simulink library "commdigbbnd"  (Simulink 5.0)
undefined symbols (not defined in the file or in its folder): j
libraries: commanabbnd x8, commutil x5, commdigbbnd x2
settings Model: Creator=tdelve  LastModifiedBy=mmclerno

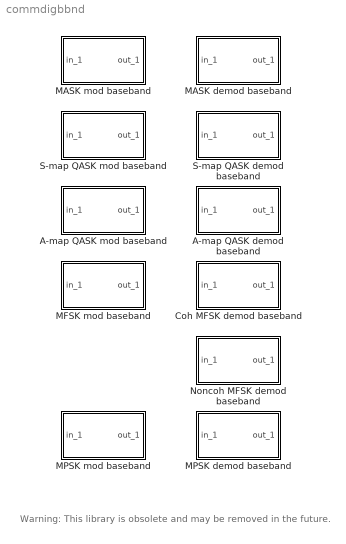
== system commdigbbnd ==
  note: Warning:  This library is obsolete and may be
      | removed in the future.
  A-map QASK demod baseband : Subsystem  mask(Baseband A-QASK demodulation){y1=real(exp(j*[0:16-1]/16*pi*2)), y2=imag(exp(j*[0:16-1]/16*pi*2)), td=0.1, num=[1;1], Ph=0, ts=0.001}
      mask prompts: y1 "Constellation in-phase component:"; y2 "Constellation quadrature component:"; td "Symbol interval and offset (sec):"; num "Lowpass filter [num; den], a 2 row matrix:"; Ph "Initial phase (rad):"; ts "Sample time (sec):"
      mask help: Demodulate the complex envelope of a QASK modulated signal. The arbitrary constellation is defined by in-phase and quadrature vectors.
      mask init:
      | den=num(2,:);num=num(1,:);
      mask Help: This block demodulates the complex envelope of a QASK modulated signal with user-defined arbitrary constellation. The vector length of the in-phase and quadrature components vectors should have the same length. The outputs are integers in the range [0, M-1], where M is the vector length of in-phase or quadrature. When the symbol interval is a two-element vector, the second element is the offset (default 0).
      mask Display:
      | plot(0,0,100,100,[5+1.5*[[0:.8:10] [10 20] [20:.8:30]] 50 50 50 50+15*[0 1 1 2 2 3]],[85+10*[sin([0:.8:10]*pi*2/5) 0 0 sin([20:.8:30]*pi*2/5)] 85 99 75 85+8*[1 1 -1 -1 1 1]]);
      | disp('A-QASK')
  A-map QASK mod baseband : Subsystem  mask(Baseband A-QASK modulation){y1=real(exp(j*[0:16-1]/16*pi*2)), y2=imag(exp(j*[0:16-1]/16*pi*2)), td=0.1, Ph=0, ts=0.001}
      mask prompts: y1 "Constellation in-phase component:"; y2 "Constellation quadrature component:"; td "Input symbol interval and offset (sec):"; Ph "Initial phase (rad):"; ts "Sample time (sec):"
      mask help: Output the complex envelope of QASK modulation. The arbitrary constellation is defined by in-phase and quadrature vectors.
      mask Help: This block outputs the complex envelope of a QASK modulated signal with user-defined arbitrary constellation. The vector length of the in-phase and quadrature components vectors should be the same length. The inputs are integers in the range [0, M-1], where M is the vector length of in-phase or quadrature. When the symbol interval is a two-element vector, the second element is the offset (default 0).
      mask Display:
      | plot(0,0,100,100,[5+15*[0 1 1 2 2 3] 50 50 50 50+1.5*[[0:.8:10] [10 20] [20:.8:30]]],[85+8*[1 1 -1 -1 1 1] 85 99 75 85+10*[sin([0:.8:10]*pi*2/5) 0 0 sin([20:.8:30]*pi*2/5)]]);
      | disp('A-QASK')
  Coh MFSK demod baseband : Subsystem  mask(Baseband coherent MFSK demodulation){M=16, Ton=16/.2/5, td=0.1, Ph=0, ts=0.001}
      mask prompts: M "M-ary number (output digits in range [0, M-1]):"; Ton "Tone space (Hz):"; td "Symbol interval (sec):"; Ph "Initial phase (rad):"; ts "Sample time (sec):"
      mask help: Demodulate the complex envelope of a MFSK modulated signal using coherent correlation method.
      mask Help: This block demodulates the complex envelope of a MFSK modulated signal using coherent method. The coherence demodulation method is phase sensitive. The tone space is the frequency distance between two successive after the modulation. The inputs are integers in the range [0, M-1], where M is the M-ary number. When the symbol interval is a two-element vector, the second element is the offset (default 0).
      mask Display:
      | plot(0,0,100,100,[5+1.5*[[0:.8:10] [10:1.6:20] [20:.8:30]] 50 50 50 50+15*[0 1 1 2 2 3]],[85+10*[sin([0:.8:10]*pi*2/5) sin([10:1.6:20]*pi/5) sin([20:.8:30]*pi*2/5)] 85 99 75 85+8*[1 1 -1 -1 1 1]]);
      | disp(' Co-MFSK')
  MASK demod baseband : Subsystem  mask(Baseband MASK demodulation){M=16, td=[.1, .1-.01], Ph=0, num=1, den=1, ts=0.001}
      mask prompts: M "M-ary number (output integer in range [0, M-1]):"; td "Output symbol interval and offset (sec):"; Ph "Initial phase (rad):"; num "Lowpass filter numerator:"; den "Lowpass filter denominator:"; ts "Filter sample time (sec):"
      mask help: Demodulate the complex envelope of a MASK modulated signal.
      mask Help: This block demodulates the complex envelope of a MASK modulated signal. The output signal are digits in the range [0, M-1]. When the output symbol interval is a two-element vector, the second element is the offset (default 0). A lowpass filter is required in the demodulation. You can set both numerator and denominator to one for not using the lowpass filter.
      mask Display:
      | plot(0,0,100,100,[5+1.5*[[0:.8:10] [10 20] [20:.8:30]] 50 50 50 50+15*[0 1 1 2 2 3]],[85+10*[sin([0:.8:10]*pi*2/5) 0 0 sin([20:.8:30]*pi*2/5)] 85 99 75 85+8*[1 1 -1 -1 1 1]]);
      | disp('MASK')
  MASK mod baseband : Subsystem  mask(Baseband MASK modulation){M=16, td=0.1, Ph=0}
      mask prompts: M "M-ary number (input integers in the range [0, M-1]):"; td "Input symbol interval and offset (sec):"; Ph "Initial phase (rad):"
      mask help: Output the complex envelope of the amplitude shift keying modulated signal.
      mask Help: This block outputs the complex envelope of MASK modulated signal. The inputs are integers in the range [0, M-1], where M is the M-ary number. The maximum amplitude of the output is 1. When the symbol interval is a two-element vector, the second element is the offset (default 0). The block takes the input value at the sampling time point.
      mask Display:
      | plot(0,0,100,100,[5+15*[0 1 1 2 2 3] 50 50 50 50+1.5*[[0:.8:10] [10 20] [20:.8:30]]],[85+8*[1 1 -1 -1 1 1] 85 99 75 85+10*[sin([0:.8:10]*pi*2/5) 0 0 sin([20:.8:30]*pi*2/5)]]);
      | disp('MASK')
  MFSK mod baseband : Subsystem  mask(Baseband MFSK modulation){Ton=16/.2/5, td=0.1, Ph=0, ts=0.001}
      mask prompts: Ton "Tone space(Hz):"; td "Symbol interval (sec):"; Ph "Initial phase (rad):"; ts "Sample time (sec):"
      mask help: Output the complex envelope of the multiple-frequency shift keying modulation.
      mask init:
      | if isinf(td),td=realmax;end;
      mask Help: This block outputs the complex envelop of MFSK modulated signal. The input signal is integers in the range [0, M-1]. The maximum amplitude of the output is 1. When the symbol interval is a two-element vector, the second element is the offset (default 0). The block takes the input value at the sampling time point.
      mask Display:
      | plot(0,0,100,100,[5+15*[0 1 1 2 2 3] 50 50 50 50+1.5*[[0:.8:10] [10:1.6:20] [20:.8:30]]],[85+8*[1 1 -1 -1 1 1] 85 99 75 85+10*[sin([0:.8:10]*pi*2/5) sin([10:1.6:20]*pi/5) sin([20:.8:30]*pi*2/5)]]);
      | disp('MFSK')
  MPSK demod baseband : Subsystem  mask(Baseband MPSK demodulation){M=16, td=0.1, Ph=0, ts=0.001}
      mask prompts: M "M-ary number (integer in range [0, M-1]):"; td "Symbol interval and offset (sec):"; Ph "Initial phase (rad):"; ts "Sample time (sec):"
      mask help: Demodulate the complex envelope of a MPSK modulated signal.
      mask Help: This block outputs the complex envelope of a MPSK modulated signal using correlation method. The output signal are digits in the range [0, M-1], where M is the M-ary number. When the symbol interval is a two-element vector, the second element is the offset (default 0).
      mask Display:
      | plot(0,0,100,100,[5+1.5*[[0:.8:10] [10:1.6:20] [20:.8:30]] 50 50 50 50+15*[0 1 1 2 2 3]],[85+10*[sin([0:.8:10]*pi*2/5) sin([10:1.6:20]*pi/5) sin([20:.8:30]*pi*2/5)] 85 99 75 85+8*[1 1 -1 -1 1 1]]);
      | disp('MPSK')
  MPSK mod baseband : Subsystem  mask(Baseband MPSK modulation){M=16, td=0.1, Ph=0}
      mask prompts: M "M-ary number (input integers in the range [0, M-1]):"; td "Symbol interval and offset (sec):"; Ph "Initial phase (rad):"
      mask help: Output the complex envelope of the M-ary phase shift keying modulation.
      mask Help: This block outputs the complex envelope of MPSK modulated signal. The inputs are integers in the range [0, M-1], where M is the M-ary number. When the symbol interval is a two-element vector, the second element is the offset (default 0). The block keeps a same input value in the symbol interval.
      mask Display:
      | plot(0,0,100,100,[5+15*[0 1 1 2 2 3] 50 50 50 50+1.5*[[0:.8:10] [10:1.6:20] [20:.8:30]]],[85+8*[1 1 -1 -1 1 1] 85 99 75 85+10*[sin([0:.8:10]*pi*2/5) sin([10:1.6:20]*pi/5) sin([20:.8:30]*pi*2/5)]]);
      | disp('MPSK')
  Noncoh MFSK demod baseband : Subsystem  mask(Baseband noncoherent MFSK demodulation){M=16, Ton=18/.2/5, td=0.1, Ph=0, ts=0.001}
      mask prompts: M "M-ary number (output digits in range [0, M-1]):"; Ton "Tone space (Hz):"; td "Symbol interval (sec):"; Ph "Initial phase (rad):"; ts "Sample time (sec):"
      mask help: Demodulate the complex envelope of a MFSK modulated signal using noncoherent correlation method.
      mask Help: This block demodulates the complex envelope of a MFSK modulated signal using noncoherent method. The coherence demodulation method is phase insensitive. The tone space is the frequency distance between two successive after the modulation. The inputs are integers in the range [0, M-1], where M is the M-ary number. When the symbol interval is a two element vector, the second element is the offset (default 0).
      mask Display:
      | plot(0,0,100,100,[5+1.5*[[0:.8:10] [10:1.6:20] [20:.8:30]] 50 50 50 50+15*[0 1 1 2 2 3]],[85+10*[sin([0:.8:10]*pi*2/5) sin([10:1.6:20]*pi/5) sin([20:.8:30]*pi*2/5)] 85 99 75 85+8*[1 1 -1 -1 1 1]]);
      | disp(' NC-MFSK')
  S-map QASK demod baseband : Subsystem  mask(Baseband S-QASK demodulation){M=16, td=0.1, num=1, den=1, Ph=0, ts=0.001}
      mask prompts: M "M-ary number (integer in range [0 M-1]):"; td "Symbol interval and offset (sec):"; num "Lowpass filter numerator:"; den "Lowpass filter denominator:"; Ph "Initial phase (rad):"; ts "Sample time (sec):"
      mask help: Demodulate the complex envelope of a QASK modulated signal. This block uses a fixed square constellation with M-ary number M=2^K, where K is an integer.
      mask Help: This block demodulates a QASK modulated signal using square constellation. The output signals are digits in the range [0, M-1], where M is the M-ary number, M=2^K, K is an integer. When the symbol interval is a two-element vector, the second element is the offset (default 0).
      mask Display:
      | plot(0,0,100,100,[5+1.5*[[0:.8:10] [10 20] [20:.8:30]] 50 50 50 50+15*[0 1 1 2 2 3]],[85+10*[sin([0:.8:10]*pi*2/5) 0 0 sin([20:.8:30]*pi*2/5)] 85 99 75 85+8*[1 1 -1 -1 1 1]]);
      | disp('S-QASK')
  S-map QASK mod baseband : Subsystem  mask(Baseband S-QASK modulation){M=16, td=0.1, Ph=0, ts=0.001}
      mask prompts: M "M-ary number (input digits in range [0, M-1]):"; td "Symbol interval and offset (sec):"; Ph "Initial phase (rad):"; ts "Sample time (sec):"
      mask help: Output the complex envelope of the QASK modulated signal. This block uses a square constellation with M-ary number M=2^K, K is an integer.
      mask Help: This block outputs the complex envelope of a QASK modulated signal. This block uses square constellation. The inputs are integers in the range [0, M-1], where M is the M-ary number, M=2^K, and K is an integer. When the symbol interval is a two-element vector, the second element is the offset (default 0).
      mask Display:
      | plot(0,0,100,100,[5+15*[0 1 1 2 2 3] 50 50 50 50+1.5*[[0:.8:10] [10 20] [20:.8:30]]],[85+8*[1 1 -1 -1 1 1] 85 99 75 85+10*[sin([0:.8:10]*pi*2/5) 0 0 sin([20:.8:30]*pi*2/5)]]);
      | disp('S-QASK')

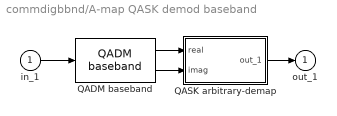
== system commdigbbnd/A-map QASK demod baseband ==
  in_1 : Inport
  QADM baseband : commanabbnd/QADM baseband  num=num  den=den  Ph=Ph  ts=ts
  QASK arbitrary-demap : Subsystem  mask(QASK A-demap){y1=y1, y2=y2, td=td}
      mask prompts: y1 "Constellation for in-phase component:"; y2 "Constellation for quadrature component:"; td "Symbol interval and offset (sec):"
      mask help: Reverse the QASK map. Input in-phase and quadrature components from the two inputs. Output demapped signal.
      mask Help: This block demaps a QASK mapped signal using user defined arbitrary constellation. You can place this block after a QAM demodulation block. The in-phase and quadrature constellation vectors must have the same length, which equals to M, the M-ary number of the QASK. The output symbols are integers in the range [0, M-1]. The symbol interval can be a two elements vector with the first element being offset. The default offset is zero.
      mask Display: disp('QASK\nA-demap')
  out_1 : Outport  InitialOutput=0
  wires:
  in_1/1 -> QADM baseband/1
  QASK arbitrary-demap/1(out_1) -> out_1/1
  QADM baseband/1 -> QASK arbitrary-demap/1(real)
  QADM baseband/2 -> QASK arbitrary-demap/2(imag)

== system commdigbbnd/A-map QASK mod baseband ==
  in_1 : Inport
  QAM baseband : commanabbnd/QAM baseband  Ph=Ph
  QASK arbitrary-map : Subsystem  mask(QASK A-map){y1=y1, y2=y2, td=td}
      mask prompts: y1 "Constellation for in-phase component:"; y2 "Constellation for quadrature component:"; td "Symbol interval and offset (sec):"
      mask help: QASK mapping for arbitrary defined map. Assume input digit is K. 1st outport outputs in-phase(K+1). 2nd outport outputs quadrature(K+1).
      mask init:
      | ly=length(y1);x=[-10 1:ly-1;1:ly-1 10*ly]-.5;x=x(:);y1=y1(:)';y1=[y1;y1];y1=y1(:);y2=y2(:)';y2=[y2;y2];y2=y2(:);
      mask Help: This block maps a digital signal onto in-phase and quadratic components, which are outputs in the first and second output port respectively. The in-phase and quadrature constellation vectors must have the same length, which equals to M, the M-ary number of the QASK. The input signal is in the range of [0, M-1]. The symbol interval can be a two elements vector with the first element being offset. The default offset is zero.
      mask Display: disp('QASK\nA-map')
  out_1 : Outport  InitialOutput=0
  wires:
  QAM baseband/1 -> out_1/1
  in_1/1 -> QASK arbitrary-map/1(in_1)
  QASK arbitrary-map/1(Real) -> QAM baseband/1
  QASK arbitrary-map/2(Imag) -> QAM baseband/2

== system commdigbbnd/Coh MFSK demod baseband ==
  in_1 : Inport
  Coh MFSK demod corr baseband : Subsystem  mask(Baseband coherent MFSK correlation){N=M, Ton=Ton, td=td, Ph=Ph, ts=ts}
      mask prompts: N "M-ary number (input in range [0, M-1]):"; Ton "Tone space (Hz):"; td "Symbol interval and offset (sec):"; Ph "Initial phase (rad):"; ts "Sample time (sec):"
      mask help: Compute baseband MFSK correlation. Take MFSK CE modulated signal. Output a vector of correlation result.
      mask init:
      | pi2=2*pi;sft=[0:N-1]*Ton*pi2;[u,v]=cmplxicn(0,50,get_param(gcb,'orientation'));
      mask Help: This block calculates the coherent correlation value of the input signal with a vector of sinusoidal signals. These sinusoidal signals have their frequency the same as that of FM modulated signal of possible resulting digits. The output is an M length vector. M is the M-ary number. The MFSK demodulation result is the index of the largest output. The computation is phase sensitive. The input of this block is complex signal.
      mask Display:
      | plot(0,0,100,100,[4 16 10 4 16 10 10 10],[54 46 50 46 54 50 58 42]);
      | disp('   Co MFSK')
  Min/max index : Subsystem  mask(Maximum/minimum index.){td=td, mima='max'}
      mask prompts: td "Symbol interval (sec):"; mima "'max' or 'min':"
      mask help: Choose the index of the input vector with max/min value at sampling point. Hold the value for the rest of the period.
      mask Help: This block outputs the index of the vector element that has the maximum or minimum value in the input vector. The computation starts at the sampling time point. The block holds the value for the rest of the interval.
      mask Display: disp('Min/Max\ndemap')
  out_1 : Outport  InitialOutput=0
  wires:
  Coh MFSK demod corr baseband/1(Out) -> Min/max index/1(in_1)
  in_1/1 -> Coh MFSK demod corr baseband/1(In)
  Min/max index/1(out_1) -> out_1/1

== system commdigbbnd/MASK demod baseband ==
  in_1 : Inport
  DSB-ADM baseband : commanabbnd/DSB-ADM baseband  num=num  den=den  Ph=Ph  ts=ts
  MASK demap : Subsystem  mask(MASK demap){M=M, td=td}
      mask prompts: M "M-ary number (output integer in range [0, M-1]):"; td "Output symbol interval and offset (sec):"
      mask help: Reverse the MASK mapping process. Convert [-1 1] analog signal to [0, M-1] symbols.
      mask init:
      | Ac=1;sft=[0:M-1]*Ac*2/(M-1)-Ac;
      mask Help: This block demaps a MASK mapped signal back to digit symbols. You can place this block after a amplitude demodulation block. The input of this block is an analog signal in the range [-1, 1]. The demodulation decides the closest integer fitting in [0,M-1] range. When the input symbol interval is a two-elements vector, the second element is offset. The default offset value is 0.
      mask Display: disp('MASK\ndemap')
  out_1 : Outport  InitialOutput=0
  wires:
  DSB-ADM baseband/1 -> MASK demap/1(in_1)
  MASK demap/1(out_1) -> out_1/1
  in_1/1 -> DSB-ADM baseband/1

== system commdigbbnd/MASK mod baseband ==
  in_1 : Inport
  DSB AM baseband : commanabbnd/DSB AM baseband  Ph=Ph
  MASK map : Subsystem  mask(MASK map){N=M, td=td}
      mask prompts: N "M-ary number (input integers in range [0, M-1]):"; td "Input symbol interval and offset (sec):"
      mask help: Map a digital symbol onto an analog signal in the range [-1, 1] using M-ary amplitude shift keying modulation mapping.
      mask init:
      | Ac=1;Kc=Ac*2/(N-1);
      mask Help: This block maps an input digit signal onto a signal in the range [-1, 1]. The coded signal can be modulated using analog\nmodulation blocks. Input digits are in the range [0, M-1], where M is the M-ary number. The input symbol interval can be a two-element vector with the second element being offset. The default value offset is 0. Use the MODMAP function to see the constellation.
      mask Display: disp('MASK\nmap')
  out_1 : Outport  InitialOutput=0
  wires:
  DSB AM baseband/1 -> out_1/1
  MASK map/1(out_1) -> DSB AM baseband/1
  in_1/1 -> MASK map/1(in_1)

== system commdigbbnd/MFSK mod baseband ==
  in_1 : Inport
  FM baseband : commanabbnd/FM baseband  Ph=Ph  HzPerV=1  ts=ts  td=td
  MFSK map : Subsystem  mask(MFSK map){Ton=Ton, td=td}
      mask prompts: Ton "Tone space (Hz):"; td "Input symbol interval and offset (sec):"
      mask help: Map input digital signal to analog tone space for FM modulation. The tone space is the frequency distance between two consective digit numbers.
      mask Help: This block maps the input digital signal to the analog signal, which is ready for the FM modulation. The input are integers in the range [0, M-1], where M is the M-ary number. Tone space is the frequency separation between two consective digits for the input signal. After FM, the modulated signal has a frequency in the range of [Fc, Fc+B]. B is the bandwidth of the FSK, B=(M-1) * Tone_space.
      mask Display: disp('MFSK\nmap')
  out_1 : Outport  InitialOutput=0
  wires:
  in_1/1 -> MFSK map/1(in_1)
  MFSK map/1(out_1) -> FM baseband/1
  FM baseband/1 -> out_1/1

== system commdigbbnd/MPSK demod baseband ==
  in_1 : Inport
  MPSK demod corr baseband : Subsystem  mask(Baseband MPSK correlationA){N=M, td=td, Ph=Ph, ts=ts}
      mask prompts: N "M-ary number (integer in range [0, M-1]):"; td "Symbol interval and offset (sec):"; Ph "Initial phase (rad):"; ts "Sample time (sec):"
      mask help: Compute Baseband MPSK correlation. Take MPSK CE modulated signal. Output a vector of correlation result.
      mask init:
      | pi2=2*pi;sft=[0:N-1]*pi2/N;
      mask Help: This block calculates the correlation value of the input signal with a vector of sinusoidal signals. These sinusoidal signals have their phase shift the same as that of PM modulated signal of possible resulting digits. The output is an M length vector. M is the M-ary number. The MPSK demodulation result is the index of the largest output, using the Min/max demap block. The input of this block is complex signal.
      mask Display: plot(0,0,100,100,[4 16 10 4 16 10 10 10],[54 46 50 46 54 50 58 42]);disp('  MPSK corr')
  Min/max index : commdigbbnd/Coh MFSK demod baseband/Min//max index  td=td  mima='max'
  out_1 : Outport  InitialOutput=0
  wires:
  MPSK demod corr baseband/1(Out) -> Min/max index/1
  in_1/1 -> MPSK demod corr baseband/1(In)
  Min/max index/1 -> out_1/1

== system commdigbbnd/MPSK mod baseband ==
  in_1 : Inport
  MPSK map : Subsystem  mask(MPSK map){td=td}
      mask prompts: td "M-ary number (input integer in range [0, M-1]):"
      mask help: Map input digital signal to analog phase shift.
      mask init:
      | pi2=2*pi;Sft=pi2/@1;
      mask Help: This block maps the input digital signal to the analog signal, which is ready for the PM modulation. The input are integers in the range [0, M-1], where M is the M-ary number. You can view the MPSK constellation using the MODMAP function.
      mask Display: disp('MPSK\nmap')
  PM baseband : commanabbnd/PM baseband  Ph=Ph  Kc=1
  out_1 : Outport  InitialOutput=0
  wires:
  MPSK map/1(out_1) -> PM baseband/1
  PM baseband/1 -> out_1/1
  in_1/1 -> MPSK map/1(in_1)

== system commdigbbnd/Noncoh MFSK demod baseband ==
  in_1 : Inport
  Min/max index : commdigbbnd/Coh MFSK demod baseband/Min//max index  td=td  mima='max'
  Non-coh MFSK dm corr baseband : Subsystem  mask(Baseband non-coherent MFSK correlation){N=M, Ton=Ton, td=td, Ph=Ph, ts=ts}
      mask prompts: N "M-ary number (input in range [0, M-1]):"; Ton "Tone space (Hz):"; td "Symbol interval and offset (sec):"; Ph "Initial phase (rad):"; ts "Sample time (sec):"
      mask help: Compute baseband MFSK correlation. Take MFSK CE modulated signal. Output a vector of correlation result.
      mask init:
      | pi2=2*pi;sft=[0:N-1]*Ton*pi2;
      mask Help: This block calculates the noncoherent correlation value of the input signal with a vector of sinusoidal signals. These sinusoidal signals have their frequency the same as that of FM modulated signal of possible resulting digits. The output is an M length vector. M is the M-ary number. The MFSK demodulation result is the index of the largest output, using the Min/max demap block. The input of this block is complex signal.
      mask Display:
      | plot(0,0,100,100, [4 16 10 4 16 10 10 10],[54 46 50 46 54 50 58 42]);
      | disp('  NC MFSK')
  out_1 : Outport  InitialOutput=0
  wires:
  Non-coh MFSK dm corr baseband/1(Out) -> Min/max index/1
  in_1/1 -> Non-coh MFSK dm corr baseband/1(In)
  Min/max index/1 -> out_1/1

== system commdigbbnd/S-map QASK demod baseband ==
  in_1 : Inport
  QADM baseband : commanabbnd/QADM baseband  num=num  den=den  Ph=Ph  ts=ts
  QASK square-demap : Subsystem  mask(QASK S-demap){N=M, td=td}
      mask prompts: N "QASK M-ary number (outputs are in range [0, M-1]):"; td "Output symbol interval and offset (sec):"
      mask help: Reverse the QASK map. Input in-phase and quadrature components from the two inputs. Output demapped signal.
      mask init:
      | Ac=1;K=log(N)/log(2);tab=flipud(constlay(K));[leny,lenx]=size(tab);sftx=[1:lenx]*2-lenx-1;sfty=[1:leny]*2-leny-1;xx=max(sftx);sftx=sftx/((xx==0)+xx)*Ac;yy=max(sfty);sfty=sfty/((yy==0)+yy)*Ac;x=[1:length(sftx)];y=[1:length(sfty)];
      | if length(y)==1, y=[y;2*y];tab=[tab;tab];end;
      mask Help: This block demaps a QASK mapped signal using square constellation. You can place this block after a QAM demodulation block. This block assumes the maximum amplitude of the input signals is 1. The output symbols are integers in the range [0, M-1]. The input symbol interval can be a two-element vector with the second element being offset. The default value offset is 0.
      mask Display: disp('QASK\nS-demap')
  out_1 : Outport  InitialOutput=0
  wires:
  QADM baseband/1 -> QASK square-demap/1(in_1)
  QADM baseband/2 -> QASK square-demap/2(in_2)
  QASK square-demap/1(out_1) -> out_1/1
  in_1/1 -> QADM baseband/1

== system commdigbbnd/S-map QASK mod baseband ==
  in_1 : Inport
  QAM baseband : commanabbnd/QAM baseband  Ph=Ph
  QASK square-map : Subsystem  mask(QASK S-map){N=M, td=td}
      mask prompts: N "M-ary number (input integers in range [0, M-1]):"; td "Input symbol interval and offset (sec):"
      mask help: Use square constellation to map the input digital signal into in-phase and quadrature components. M must be M=2^K with integer K.
      mask init:
      | Ac=1;z=[[1:N];[1:N]];z=z(:);[x,y]=qaskenco(z-1,N);z=z-1.5;z=[z(2:2*N);N-.5];xx=max(x);yy=max(y);x=x/((xx==0)+xx);y=y/((yy==0)+yy);
      mask Help: This block maps a digital signal onto in-phase and quadratic components, which are outputs in the first and second output port respectively. The M-ary number must be M=2^K with integer K. The input symbol interval can be a two-element vector with the second element being offset. The default value offset is 0. The maximum amplitudes for the outputs are 1.
      mask Display: disp('QASK\nS-map')
  out_1 : Outport  InitialOutput=0
  wires:
  QASK square-map/1(out_1) -> QAM baseband/1
  QASK square-map/2(out_2) -> QAM baseband/2
  QAM baseband/1 -> out_1/1
  in_1/1 -> QASK square-map/1(in_1)

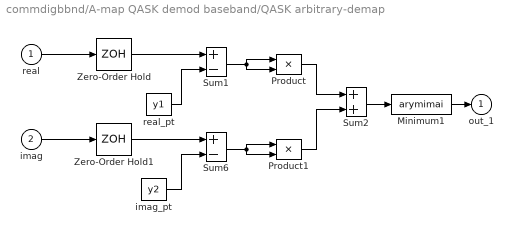
== system commdigbbnd/A-map QASK demod baseband/QASK arbitrary-demap ==
  real : Inport
  imag : Inport  Port=2
  Minimum1 : S-Function  FunctionName=arymimai  Parameters='min'
  Product : Product  SaturateOnIntegerOverflow=on  InputSameDT=on
  Product1 : Product  SaturateOnIntegerOverflow=on  InputSameDT=on
  Sum1 : Sum  Inputs=+-  SaturateOnIntegerOverflow=on  InputSameDT=on
  Sum2 : Sum  SaturateOnIntegerOverflow=on  InputSameDT=on
  Sum6 : Sum  Inputs=+-  SaturateOnIntegerOverflow=on  InputSameDT=on
  Zero-Order Hold : ZeroOrderHold  SampleTime=td
  Zero-Order Hold1 : ZeroOrderHold  SampleTime=td
  imag_pt : Constant  Value=y2
  real_pt : Constant  Value=y1
  out_1 : Outport  InitialOutput=0
  wires:
  Minimum1/1 -> out_1/1
  Sum2/1 -> Minimum1/1
  Product1/1 -> Sum2/2
  Product/1 -> Sum2/1
  Sum6/1 -> Product1/1, Product1/2
  Sum1/1 -> Product/1, Product/2
  imag_pt/1 -> Sum6/2
  Zero-Order Hold1/1 -> Sum6/1
  Zero-Order Hold/1 -> Sum1/1
  real_pt/1 -> Sum1/2
  imag/1 -> Zero-Order Hold1/1
  real/1 -> Zero-Order Hold/1

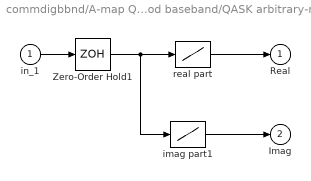
== system commdigbbnd/A-map QASK mod baseband/QASK arbitrary-map ==
  in_1 : Inport
  Zero-Order Hold1 : ZeroOrderHold  SampleTime=td
  imag part1 : Lookup  InputValues=x  OutputValues=y2  SaturateOnIntegerOverflow=on
  real part : Lookup  InputValues=x  OutputValues=y1  SaturateOnIntegerOverflow=on
  Real : Outport  InitialOutput=0
  Imag : Outport  Port=2  InitialOutput=0
  wires:
  imag part1/1 -> Imag/1
  real part/1 -> Real/1
  Zero-Order Hold1/1 -> real part/1, imag part1/1
  in_1/1 -> Zero-Order Hold1/1

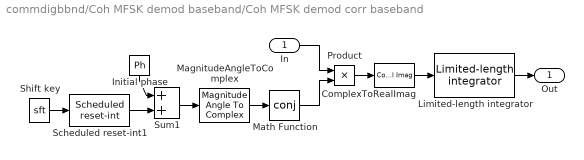
== system commdigbbnd/Coh MFSK demod baseband/Coh MFSK demod corr baseband ==
  In : Inport
  ComplexToRealImag : ComplexToRealImag  Output=Real
  Initial phase : Constant  Orientation=down  Value=Ph
  Limited-length integrator : commutil/Limited-length integrator  vec=N  T=td  sample_time=ts  method='backward'
  MagnitudeAngleToComplex : MagnitudeAngleToComplex  Input=Angle  ConstantPart=1
  Math Function : Math  Operator=conj
  Product : Product  SaturateOnIntegerOverflow=on  InputSameDT=on
  Scheduled reset-int1 : commutil/Scheduled reset-int  td=td  ts=ts  limit=Inf
  Shift key : Constant  Value=sft
  Sum1 : Sum  SaturateOnIntegerOverflow=on  InputSameDT=on
  Out : Outport  InitialOutput=0
  wires:
  Limited-length integrator/1 -> Out/1
  ComplexToRealImag/1 -> Limited-length integrator/1
  Product/1 -> ComplexToRealImag/1
  Initial phase/1 -> Sum1/1
  Shift key/1 -> Scheduled reset-int1/1
  Scheduled reset-int1/1 -> Sum1/2
  In/1 -> Product/1
  Math Function/1 -> Product/2
  MagnitudeAngleToComplex/1 -> Math Function/1
  Sum1/1 -> MagnitudeAngleToComplex/1

== system commdigbbnd/Coh MFSK demod baseband/Min/max index ==
  in_1 : Inport
  Maximum : S-Function  FunctionName=arymimai  Parameters=mima
  Zero-Order Hold : ZeroOrderHold  SampleTime=td
  out_1 : Outport  InitialOutput=0
  wires:
  Zero-Order Hold/1 -> Maximum/1
  Maximum/1 -> out_1/1
  in_1/1 -> Zero-Order Hold/1

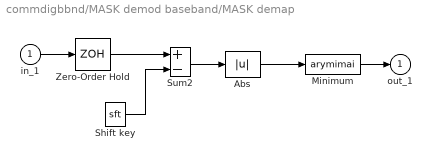
== system commdigbbnd/MASK demod baseband/MASK demap ==
  in_1 : Inport
  Abs : Abs  SaturateOnIntegerOverflow=on
  Minimum : S-Function  FunctionName=arymimai  Parameters='min'
  Shift key : Constant  Value=sft
  Sum2 : Sum  Inputs=+-  SaturateOnIntegerOverflow=on  InputSameDT=on
  Zero-Order Hold : ZeroOrderHold  SampleTime=td
  out_1 : Outport  InitialOutput=0
  wires:
  Sum2/1 -> Abs/1
  Shift key/1 -> Sum2/2
  Minimum/1 -> out_1/1
  Zero-Order Hold/1 -> Sum2/1
  Abs/1 -> Minimum/1
  in_1/1 -> Zero-Order Hold/1

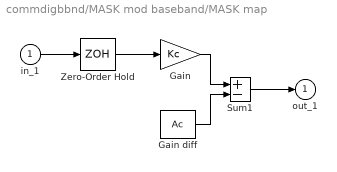
== system commdigbbnd/MASK mod baseband/MASK map ==
  in_1 : Inport
  Gain : Gain  Gain=Kc  SaturateOnIntegerOverflow=on
  Gain diff : Constant  Value=Ac
  Sum1 : Sum  Inputs=+-  SaturateOnIntegerOverflow=on  InputSameDT=on
  Zero-Order Hold : ZeroOrderHold  SampleTime=td
  out_1 : Outport  InitialOutput=0
  wires:
  Zero-Order Hold/1 -> Gain/1
  in_1/1 -> Zero-Order Hold/1
  Sum1/1 -> out_1/1
  Gain diff/1 -> Sum1/2
  Gain/1 -> Sum1/1

== system commdigbbnd/MFSK mod baseband/MFSK map ==
  in_1 : Inport
  Gain : Gain  Gain=Ton  SaturateOnIntegerOverflow=on
  Zero-Order Hold1 : ZeroOrderHold  SampleTime=td
  out_1 : Outport  InitialOutput=0
  wires:
  Gain/1 -> out_1/1
  in_1/1 -> Zero-Order Hold1/1
  Zero-Order Hold1/1 -> Gain/1

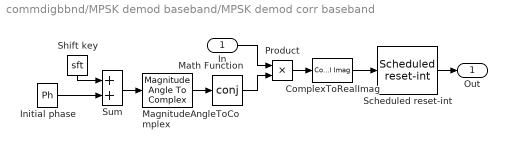
== system commdigbbnd/MPSK demod baseband/MPSK demod corr baseband ==
  In : Inport
  ComplexToRealImag : ComplexToRealImag  Output=Real
  Initial phase : Constant  Value=Ph
  MagnitudeAngleToComplex : MagnitudeAngleToComplex  Input=Angle  ConstantPart=1
  Math Function : Math  Operator=conj
  Product : Product  SaturateOnIntegerOverflow=on  InputSameDT=on
  Scheduled reset-int : commutil/Scheduled reset-int  td=td  ts=ts  limit=Inf
  Shift key : Constant  Orientation=down  Value=sft
  Sum : Sum  SaturateOnIntegerOverflow=on  InputSameDT=on
  Out : Outport  InitialOutput=0
  wires:
  Scheduled reset-int/1 -> Out/1
  ComplexToRealImag/1 -> Scheduled reset-int/1
  In/1 -> Product/1
  Math Function/1 -> Product/2
  Product/1 -> ComplexToRealImag/1
  Sum/1 -> MagnitudeAngleToComplex/1
  MagnitudeAngleToComplex/1 -> Math Function/1
  Shift key/1 -> Sum/1
  Initial phase/1 -> Sum/2

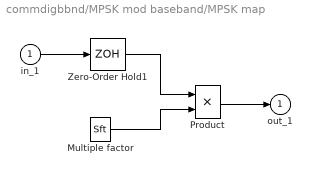
== system commdigbbnd/MPSK mod baseband/MPSK map ==
  in_1 : Inport
  Multiple factor : Constant  Value=Sft
  Product : Product  SaturateOnIntegerOverflow=on  InputSameDT=on
  Zero-Order Hold1 : ZeroOrderHold  SampleTime=td
  out_1 : Outport  InitialOutput=0
  wires:
  Multiple factor/1 -> Product/2
  Product/1 -> out_1/1
  in_1/1 -> Zero-Order Hold1/1
  Zero-Order Hold1/1 -> Product/1

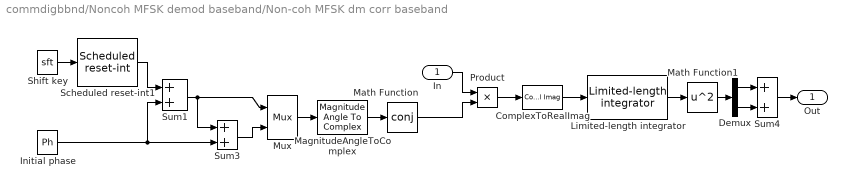
== system commdigbbnd/Noncoh MFSK demod baseband/Non-coh MFSK dm corr baseband ==
  In : Inport
  ComplexToRealImag : ComplexToRealImag  Output=Real
  Demux : Demux  Outputs=2
  Initial phase : Constant  Value=Ph
  Limited-length integrator : commutil/Limited-length integrator  vec=N*2  T=td  sample_time=ts  method='backward'
  MagnitudeAngleToComplex : MagnitudeAngleToComplex  Input=Angle  ConstantPart=1
  Math Function : Math  Operator=conj
  Math Function1 : Math  Operator=square
  Mux : Mux  Inputs=2
  Product : Product  SaturateOnIntegerOverflow=on  InputSameDT=on
  Scheduled reset-int1 : commutil/Scheduled reset-int  td=td  ts=ts  limit=Inf
  Shift key : Constant  Value=sft
  Sum1 : Sum  SaturateOnIntegerOverflow=on  InputSameDT=on
  Sum3 : Sum  SaturateOnIntegerOverflow=on  InputSameDT=on
  Sum4 : Sum  SaturateOnIntegerOverflow=on  InputSameDT=on
  Out : Outport  InitialOutput=0
  wires:
  Demux/1 -> Sum4/1
  Demux/2 -> Sum4/2
  Limited-length integrator/1 -> Math Function1/1
  Sum4/1 -> Out/1
  Math Function1/1 -> Demux/1
  ComplexToRealImag/1 -> Limited-length integrator/1
  Product/1 -> ComplexToRealImag/1
  MagnitudeAngleToComplex/1 -> Math Function/1
  Math Function/1 -> Product/2
  In/1 -> Product/1
  Mux/1 -> MagnitudeAngleToComplex/1
  Sum3/1 -> Mux/2
  Shift key/1 -> Scheduled reset-int1/1
  Scheduled reset-int1/1 -> Sum1/1
  Sum1/1 -> Sum3/1, Mux/1
  Initial phase/1 -> Sum3/2, Sum1/2

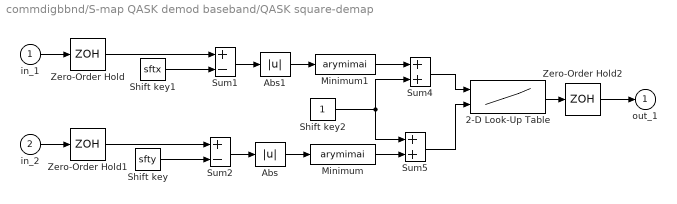
== system commdigbbnd/S-map QASK demod baseband/QASK square-demap ==
  in_1 : Inport
  in_2 : Inport  Port=2
  2-D Look-Up Table : Lookup2D  RowIndex=x  ColumnIndex=y  OutputValues=tab'  SaturateOnIntegerOverflow=on  InputSameDT=on
  Abs : Abs  SaturateOnIntegerOverflow=on
  Abs1 : Abs  SaturateOnIntegerOverflow=on
  Minimum : S-Function  FunctionName=arymimai  Parameters='min'
  Minimum1 : S-Function  FunctionName=arymimai  Parameters='min'
  Shift key : Constant  Value=sfty
  Shift key1 : Constant  Value=sftx
  Shift key2 : Constant
  Sum1 : Sum  Inputs=+-  SaturateOnIntegerOverflow=on  InputSameDT=on
  Sum2 : Sum  Inputs=+-  SaturateOnIntegerOverflow=on  InputSameDT=on
  Sum4 : Sum  SaturateOnIntegerOverflow=on  InputSameDT=on
  Sum5 : Sum  SaturateOnIntegerOverflow=on  InputSameDT=on
  Zero-Order Hold : ZeroOrderHold  SampleTime=td
  Zero-Order Hold1 : ZeroOrderHold  SampleTime=td
  Zero-Order Hold2 : ZeroOrderHold  SampleTime=td
  out_1 : Outport  InitialOutput=0
  wires:
  Shift key1/1 -> Sum1/2
  Sum1/1 -> Abs1/1
  Abs1/1 -> Minimum1/1
  Sum4/1 -> 2-D Look-Up Table/1
  Minimum1/1 -> Sum4/1
  Zero-Order Hold/1 -> Sum1/1
  Shift key2/1 -> Sum4/2, Sum5/1
  Sum5/1 -> 2-D Look-Up Table/2
  Minimum/1 -> Sum5/2
  Zero-Order Hold1/1 -> Sum2/1
  Shift key/1 -> Sum2/2
  Sum2/1 -> Abs/1
  Abs/1 -> Minimum/1
  Zero-Order Hold2/1 -> out_1/1
  2-D Look-Up Table/1 -> Zero-Order Hold2/1
  in_1/1 -> Zero-Order Hold/1
  in_2/1 -> Zero-Order Hold1/1

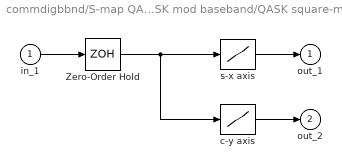
== system commdigbbnd/S-map QASK mod baseband/QASK square-map ==
  in_1 : Inport
  Zero-Order Hold : ZeroOrderHold  SampleTime=td
  c-y axis : Lookup  InputValues=z  OutputValues=y  SaturateOnIntegerOverflow=on
  s-x axis : Lookup  InputValues=z  OutputValues=x  SaturateOnIntegerOverflow=on
  out_1 : Outport  InitialOutput=0
  out_2 : Outport  Port=2  InitialOutput=0
  wires:
  in_1/1 -> Zero-Order Hold/1
  Zero-Order Hold/1 -> s-x axis/1, c-y axis/1
  c-y axis/1 -> out_2/1
  s-x axis/1 -> out_1/1
